simulink model "A2_Part3_simulink_model"  (R2019a)
settings: Solver=FixedStepAuto  StartTime=0.0  StopTime=1000  FixedStep=0.01  RelTol=1e-3
values from neighbouring files (symbols this model uses):
  k_i_chi = omega_n_chi^2 * V_g/g    [A2_Part2.m]
  k_i_phi = 0.0    (= 0)    [A2_Part2.m]
  k_p_chi = 2 * zeta_chi * omega_n_chi * V_g/g    [A2_Part2.m]
  k_p_phi = delta_a_max/e_phi_max * sign(a_phi_2)    [A2_Part2.m]
  V_g = V_a    [A2_Part2.m]
undefined symbols (not defined in the file or in its folder): chi_ref, g
libraries: simulink_extras x13, dspsrcs4 x2
settings Model: Creator=paalthorseth  LastModifiedBy=gustavoo

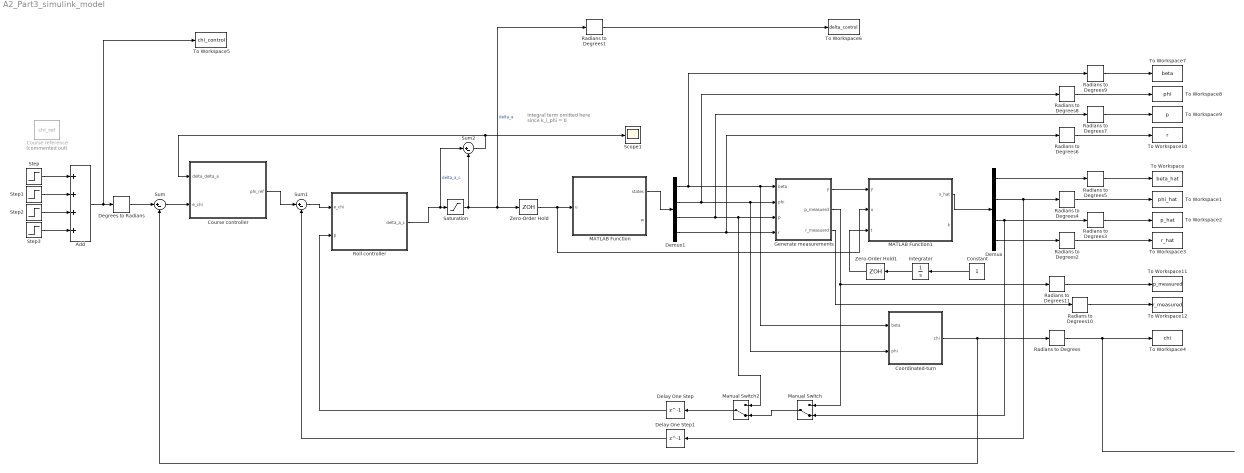
== system A2_Part3_simulink_model ==
  note: Integral term omitted here
      | since k_i_phi = 0
  Add : Sum  Inputs=++++
  Constant : Constant
  Coordinated-turn : Subsystem
  "Course controller " : Subsystem
  "Course reference " : Constant  Commented=on  Value=chi_ref
  Degrees to Radians : simulink_extras/Transformations/Degrees to Radians
  Delay One Step : Delay  DelayLength=1
  Delay One Step1 : Delay  DelayLength=1
  Demux : Demux
  Demux1 : Demux
  Generate measurements : Subsystem
  Integrator : Integrator
  MATLAB Function : MATLAB Function  TreatAsAtomicUnit=on
  MATLAB Function1 : MATLAB Function  TreatAsAtomicUnit=on
  Manual Switch : ManualSwitch  CurrentSetting=0
  Manual Switch2 : ManualSwitch  CurrentSetting=0
  Radians to Degrees{,1..11} (12 alike) : simulink_extras/Transformations/Radians to Degrees
  Roll controller : Subsystem
  Saturation : Saturate  UpperLimit=pi/6  LowerLimit=-pi/6
  Scope1 : Scope
  Step : Step  Time=100  After=7.5  SampleTime=0
  Step1 : Step  Time=150  After=7.5  SampleTime=0
  Step2 : Step  Time=250  After=-15  SampleTime=0
  Step3 : Step  Time=300  After=-5  SampleTime=0
  Sum : Sum  Inputs=|+-
  Sum1 : Sum  Inputs=|+-
  Sum2 : Sum  Inputs=|+-
  To Workspace : ToWorkspace  VariableName=beta_hat  SaveFormat=Timeseries  SampleTime=-1
  To Workspace1 : ToWorkspace  VariableName=phi_hat  SaveFormat=Timeseries  SampleTime=-1
  To Workspace10 : ToWorkspace  VariableName=r  SaveFormat=Timeseries  SampleTime=-1
  To Workspace11 : ToWorkspace  VariableName=p_measured  SaveFormat=Timeseries  SampleTime=-1
  To Workspace12 : ToWorkspace  VariableName=r_measured  SaveFormat=Timeseries  SampleTime=-1
  To Workspace2 : ToWorkspace  VariableName=p_hat  SaveFormat=Timeseries  SampleTime=-1
  To Workspace3 : ToWorkspace  VariableName=r_hat  SaveFormat=Timeseries  SampleTime=-1
  To Workspace4 : ToWorkspace  VariableName=chi  SaveFormat=Timeseries  SampleTime=-1
  To Workspace5 : ToWorkspace  VariableName=chi_control  SaveFormat=Timeseries  SampleTime=-1
  To Workspace6 : ToWorkspace  VariableName=delta_control  SaveFormat=Timeseries  SampleTime=-1
  To Workspace7 : ToWorkspace  VariableName=beta  SaveFormat=Timeseries  SampleTime=-1
  To Workspace8 : ToWorkspace  VariableName=phi  SaveFormat=Timeseries  SampleTime=-1
  To Workspace9 : ToWorkspace  VariableName=p  SaveFormat=Timeseries  SampleTime=-1
  Zero-Order Hold : ZeroOrderHold  SampleTime=-1
  Zero-Order Hold1 : ZeroOrderHold  SampleTime=-1
  wires:
  Coordinated-turn/1(chi) -> Radians to Degrees/1, Sum/2
  "Course controller "/1("phi_ref ") -> Sum1/1
  Delay One Step1/1 -> Sum1/2
  Sum1/1 -> Roll controller/1(e_chi)
  Delay One Step/1 -> Roll controller/2(p)
  Zero-Order Hold/1 -> MATLAB Function1/2(u), MATLAB Function/1(u)
  Generate measurements/1(y) -> MATLAB Function1/1(y)
  MATLAB Function1/1(x_hat) -> Demux/1
  Demux/1 -> Radians to Degrees5/1
  Demux/2 -> Delay One Step1/1, Radians to Degrees4/1
  Demux/4 -> Radians to Degrees2/1
  Demux/3 -> Manual Switch/2, Radians to Degrees3/1
  MATLAB Function/1(states) -> Demux1/1
  Demux1/2 -> Generate measurements/2(phi), Coordinated-turn/2(phi), Radians to Degrees8/1
  Demux1/3 -> Radians to Degrees7/1, Manual Switch2/1, Generate measurements/3(p)
  Demux1/4 -> Radians to Degrees6/1, Generate measurements/4(r)
  Demux1/1 -> Coordinated-turn/1(beta), Generate measurements/1("beta "), Radians to Degrees9/1
  Step2/1 -> Add/3
  Step3/1 -> Add/4
  Step1/1 -> Add/2
  Step/1 -> Add/1
  Degrees to Radians/1 -> Sum/1
  Constant/1 -> Integrator/1
  Integrator/1 -> Zero-Order Hold1/1
  Zero-Order Hold1/1 -> MATLAB Function1/3(t)
  Generate measurements/2(p_measuerd) -> Manual Switch/1, Radians to Degrees11/1
  Radians to Degrees/1 -> To Workspace4/1
  Saturation/1 -> Sum2/2, Radians to Degrees1/1, Zero-Order Hold/1  "delta_a"
  Roll controller/1("delta_a_c ") -> Sum2/1, Saturation/1  "delta_a_c"
  Sum/1 -> "Course controller "/2(e_chi)
  Sum2/1 -> "Course controller "/1("delta_delta_a "), Scope1/1
  Add/1 -> To Workspace5/1, Degrees to Radians/1
  Radians to Degrees1/1 -> To Workspace6/1
  Radians to Degrees2/1 -> To Workspace3/1
  Radians to Degrees3/1 -> To Workspace2/1
  Radians to Degrees4/1 -> To Workspace1/1
  Radians to Degrees5/1 -> To Workspace/1
  Radians to Degrees6/1 -> To Workspace10/1
  Radians to Degrees7/1 -> To Workspace9/1
  Radians to Degrees8/1 -> To Workspace8/1
  Radians to Degrees9/1 -> To Workspace7/1
  Radians to Degrees10/1 -> To Workspace12/1
  Radians to Degrees11/1 -> To Workspace11/1
  Generate measurements/3(r_measuerd) -> Radians to Degrees10/1
  Manual Switch/1 -> Manual Switch2/2
  Manual Switch2/1 -> Delay One Step/1

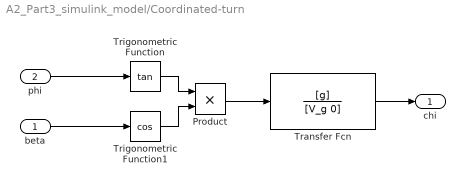
== system A2_Part3_simulink_model/Coordinated-turn ==
  beta : Inport
  phi : Inport  Port=2
  Product : Product
  Transfer Fcn : TransferFcn  Numerator=[g]  Denominator=[V_g 0]
  Trigonometric Function : Trigonometry  Operator=tan
  Trigonometric Function1 : Trigonometry  Operator=cos
  chi : Outport
  wires:
  phi/1 -> Trigonometric Function/1
  beta/1 -> Trigonometric Function1/1
  Trigonometric Function/1 -> Product/1
  Trigonometric Function1/1 -> Product/2
  Transfer Fcn/1 -> chi/1
  Product/1 -> Transfer Fcn/1

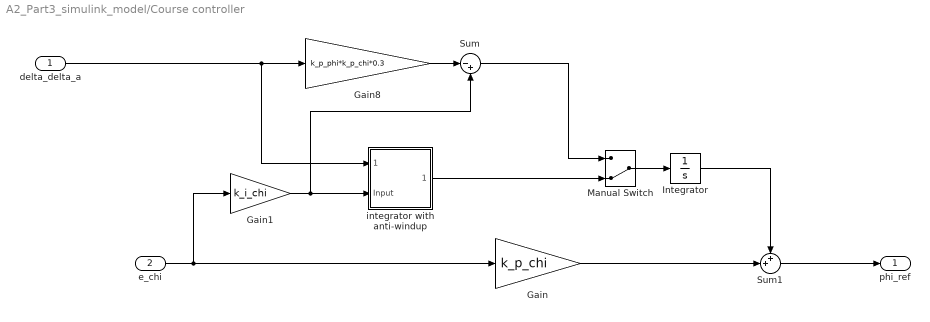
== system A2_Part3_simulink_model/Course controller  ==
  "delta_delta_a " : Inport
  e_chi : Inport  Port=2
  Gain : Gain  Gain=k_p_chi
  Gain1 : Gain  Gain=k_i_chi
  Gain8 : Gain  Gain=k_p_phi*k_p_chi*0.3
  Integrator : Integrator
  Manual Switch : ManualSwitch  CurrentSetting=0
  Sum : Sum  Inputs=|-+
  Sum1 : Sum  Inputs=++|
  integrator with anti-windup : Subsystem
  "phi_ref " : Outport
  wires:
  Sum1/1 -> "phi_ref "/1
  e_chi/1 -> Gain/1, Gain1/1
  Gain/1 -> Sum1/2
  Gain1/1 -> Sum/2, integrator with anti-windup/2(Input)
  "delta_delta_a "/1 -> integrator with anti-windup/1(delta_a), Gain8/1
  Manual Switch/1 -> Integrator/1
  Sum/1 -> Manual Switch/1
  integrator with anti-windup/1(Output) -> Manual Switch/2
  Integrator/1 -> Sum1/1
  Gain8/1 -> Sum/1

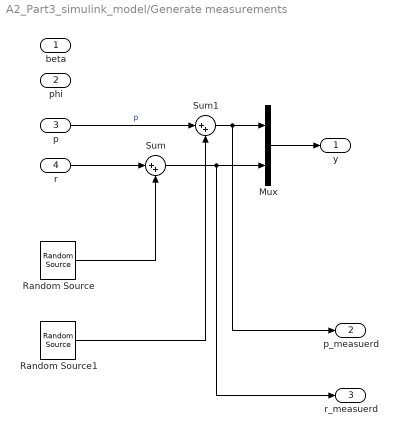
== system A2_Part3_simulink_model/Generate measurements ==
  "beta " : Inport
  phi : Inport  Port=2
  p : Inport  Port=3
  r : Inport  Port=4
  Mux : Mux  Inputs=2
  Random Source : dspsrcs4/Random Source  SrcType=Gaussian  NormMethod=Ziggurat  CltLength=12  MinVal=0  MaxVal=1  MeanVal=0  VarVal=(0.2*pi/180)^2  RepMode=Not repeatable  rawSeed=1  IsInherit=off  SampMode=Discrete  SampTime=0.01  SampFrame=1  DataType=Double  OutComplex=Real  OutputFrames=off
  Random Source1 : dspsrcs4/Random Source  SrcType=Gaussian  NormMethod=Ziggurat  CltLength=12  MinVal=0  MaxVal=1  MeanVal=0  VarVal=(0.2*pi/180)^2  RepMode=Not repeatable  rawSeed=1  IsInherit=off  SampMode=Discrete  SampTime=0.01  SampFrame=1  DataType=Double  OutComplex=Real  OutputFrames=off
  Sum : Sum  Inputs=|++
  Sum1 : Sum  Inputs=|++
  y : Outport
  p_measuerd : Outport  Port=2
  r_measuerd : Outport  Port=3
  wires:
  Mux/1 -> y/1
  p/1 -> Sum1/1  "p"
  r/1 -> Sum/1
  Sum/1 -> r_measuerd/1, Mux/2
  Sum1/1 -> p_measuerd/1, Mux/1
  Random Source/1 -> Sum/2
  Random Source1/1 -> Sum1/2

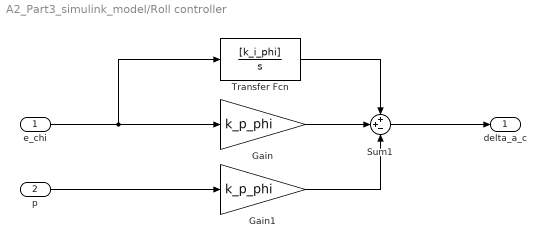
== system A2_Part3_simulink_model/Roll controller ==
  e_chi : Inport
  p : Inport  Port=2
  Gain : Gain  Gain=k_p_phi
  Gain1 : Gain  Gain=k_p_phi
  Sum1 : Sum  Inputs=++-
  Transfer Fcn : TransferFcn  Numerator=[k_i_phi]  Denominator=[1 0]
  "delta_a_c " : Outport
  wires:
  Sum1/1 -> "delta_a_c "/1
  e_chi/1 -> Gain/1, Transfer Fcn/1
  Gain/1 -> Sum1/2
  Transfer Fcn/1 -> Sum1/1
  p/1 -> Gain1/1
  Gain1/1 -> Sum1/3

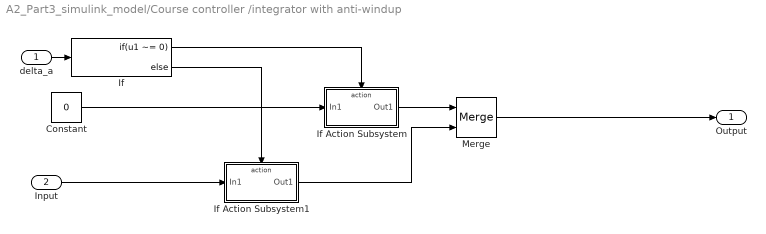
== system A2_Part3_simulink_model/Course controller /integrator with anti-windup ==
  delta_a : Inport
  Input : Inport  Port=2
  Constant : Constant  Value=0
  If : If  IfExpression=u1 ~= 0
  If Action Subsystem : Subsystem  TreatAsAtomicUnit=on
  If Action Subsystem1 : Subsystem  TreatAsAtomicUnit=on
  Merge : Merge
  Output : Outport
  wires:
  If/2 -> If Action Subsystem1/Action
  If/1 -> If Action Subsystem/Action
  If Action Subsystem1/1(Out1) -> Merge/2
  If Action Subsystem/1(Out1) -> Merge/1
  delta_a/1 -> If/1
  Constant/1 -> If Action Subsystem/1(In1)
  Input/1 -> If Action Subsystem1/1(In1)
  Merge/1 -> Output/1

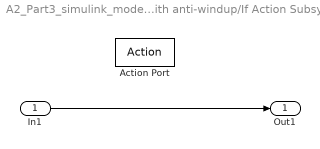
== system A2_Part3_simulink_model/Course controller /integrator with anti-windup/If Action Subsystem ==
  In1 : Inport
  Action Port : ActionPort  ActionPortLabel=if(u1 ~= 0)
  Out1 : Outport
  wires:
  In1/1 -> Out1/1

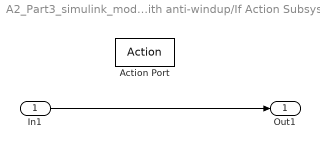
== system A2_Part3_simulink_model/Course controller /integrator with anti-windup/If Action Subsystem1 ==
  In1 : Inport
  Action Port : ActionPort  ActionPortLabel=else
  Out1 : Outport
  wires:
  In1/1 -> Out1/1

== matlab function A2_Part3_simulink_model/MATLAB Function1 ==
  data: y input; x_hat output; u input; t input; k output
function [x_hat, k]= kalman(y, u, t)
    persistent init_flag P_a_priori x_hat_a_priori P_post_priori y_a_priori S 

    if isempty(init_flag)
        S = load('kalman_variables');
        init_flag = 1;
        P_a_priori = S.P0_a_priori;
        x_hat_a_priori = S.x_hat_0_a_priori;
    end
    
    if t > 250
        S.R = [10000000 0;0 10000000];
    end
    
    kalman_gain = P_a_priori*transpose(S.C)*inv(S.C*P_a_priori*transpose(S.C)+S.R);
    P_post_priori = P_a_priori - kalman_gain*S.C*P_a_priori - P_a_priori*transpose(S.C)...
        *transpose(kalman_gain) + kalman_gain*(S.C*P_a_priori*transpose(S.C)+S.R)*transpose(kalman_gain);
    y_a_priori = S.C*x_hat_a_priori;
    x_hat = x_hat_a_priori + kalman_gain*(y - y_a_priori);
    x_hat_a_priori = S.A_d*x_hat + S.B_d*u;
    P_a_priori =  S.A_d*P_post_priori*transpose(S.A_d)+S.E_d*S.Q*transpose(S.E_d);
    k = kalman_gain;
end

== matlab function A2_Part3_simulink_model/MATLAB Function ==
  data: u input; states output; w output
function [states, w] = state_space(u)
% Generate the output of the state space

    % Persistent variables to be kept between function calls
    persistent counter; % Variable for checking if it is the first iteration.
    persistent x;       % The state x
    
   % The next line is necessary for generating unique process noise for every simulation.
   % Otherwise, the noise will be equal every time you run the simulation,
   % even though it is white. This has to do with how Matlab generates
   % random numbers. 
   coder.extrinsic('randn','rng');
    
    h = 0.01;       % Time step of Euler integration
    delta_a_c = u;  % Aileron input
    
    if isempty(counter)
      % First iteration
        counter = 1;
           
        % Initialize state space
        x = zeros(5,1);
        w = zeros(5,1); 
        rng('shuffle'); % Necessary for generating unique process noise for every simulation.
    
    else
        % State-space matrices
        A = [-0.322, 0.052, 0.028, -1.12, 0.002;
             0, 0, 1, -0.001, 0;
             -10.6, 0, -2.87, 0.46, -0.65;
             6.87, 0, -0.04, -0.32, -0.02;
             0, 0, 0, 0, -7.5];
 
        B = [0; 0; 0; 0; 7.5;];
        
        E = eye(5);
        
        % Discrete version
        Ad = eye(5) + h*A;
        Bd = h*B;
        Ed = E;
        
        % The Qd matrix in the assignment is given directly in discrete-time here and
        % therefore, it is not necessary to discretize E.
        Qd = h*10^-6*[0.001, 0, 0, 0, 0;
                  0, 1, 0, 0, 0;
                  0, 0, 100, 0, 0;
                  0, 0, 0, 10, 0;
                  0, 0, 0, 0, 0];
          
        w = sqrt(Qd)*randn(5,1,1); % The standard deviation must be multiplied with random numbers with a zero-mean unit variance random number to generate process noise. 
        
        % Discrete-time state space update
        x = Ad*x + Bd * delta_a_c + Ed*w;
    end
    states = x(1:4); % Return every state except the actuator state.
end
